simulink model "practice8_1"  (Simulink 7.9)
settings: Solver=ode45  StartTime=0.0  StopTime=35  RelTol=1e-3
settings Model: Creator=sony  LastModifiedBy=sony

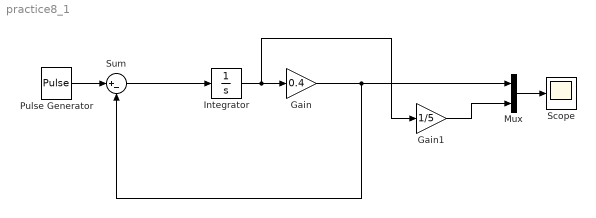
== system practice8_1 ==
  Gain : Gain  Gain=0.4
  Gain1 : Gain  Gain=1/5
  Integrator : Integrator
  Mux : Mux  Inputs=2
  Pulse Generator : DiscretePulseGenerator  PulseType=Time based  Amplitude=400/0.07  Period=7
  Scope : Scope
  Sum : Sum  Inputs=|+-
  wires:
  Pulse Generator/1 -> Sum/1
  Sum/1 -> Integrator/1
  Integrator/1 -> Gain/1, Gain1/1
  Gain/1 -> Mux/1, Sum/2
  Mux/1 -> Scope/1
  Gain1/1 -> Mux/2
